simulink model "Sim36"  (R2019a)
settings: Solver=FixedStepAuto  StartTime=0.0  StopTime=10.0  FixedStep=0.0001  RelTol=1e-3
settings Model: Creator=fbleo  LastModifiedBy=fbleo

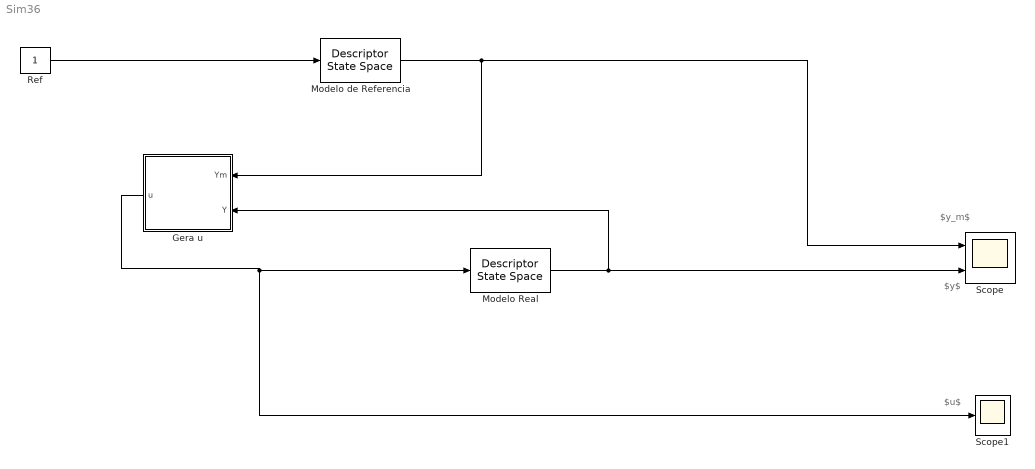
== system Sim36 ==
  note: $y$
  note: $u$
  note: $y_m$
  Gera u : Subsystem
  Modelo Real : DescriptorStateSpace  A=-1  B=2  D=0  InitialCondition=0.5
  Modelo de Referencia : DescriptorStateSpace  A=-3  B=3  D=0  InitialCondition=0
  Ref : Constant
  Scope : Scope  NumInputPorts=2
  Scope1 : Scope
  wires:
  Modelo de Referencia/1 -> Scope/1, Gera u/1(Ym)
  Modelo Real/1 -> Scope/2, Gera u/2(Y)
  Gera u/1(u) -> Modelo Real/1, Scope1/1
  Ref/1 -> Modelo de Referencia/1

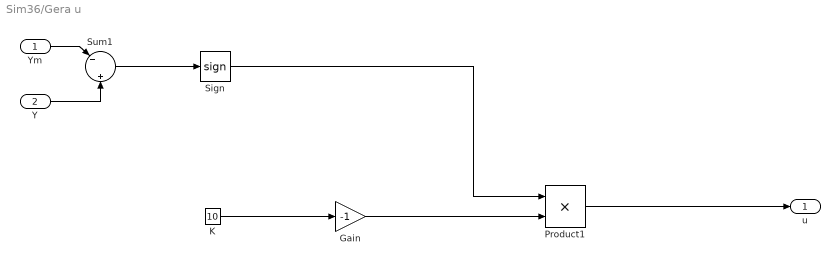
== system Sim36/Gera u ==
  Ym : Inport
  Y : Inport  Port=2
  Gain : Gain  Gain=-1
  K : Constant  Value=10
  Product1 : Product
  Sign : Signum
  Sum1 : Sum  Inputs=|-||+
  u : Outport
  wires:
  Ym/1 -> Sum1/1
  Y/1 -> Sum1/2
  Sum1/1 -> Sign/1
  Product1/1 -> u/1
  Sign/1 -> Product1/1
  Gain/1 -> Product1/2
  K/1 -> Gain/1
